simulink model "Correlation_Ex4"  (R2025a)
settings: Solver=VariableStepAuto  StartTime=0.0  StopTime=1024/100e6  RelTol=1e-3
undefined symbols (not defined in the file): Correlation_ValidMode, DUT, S, Valid, vsva2197, xcvc1902
libraries: visionstatistics x1, aieDSP x1, vmcUtilities x1
settings Model: Creator=sdegala  LastModifiedBy=robg
settings ModelReferenceCC: EnableRefExpFcnMdlSchedulingChecks=on
settings RTWCC: GPUComputeCapability=3.5

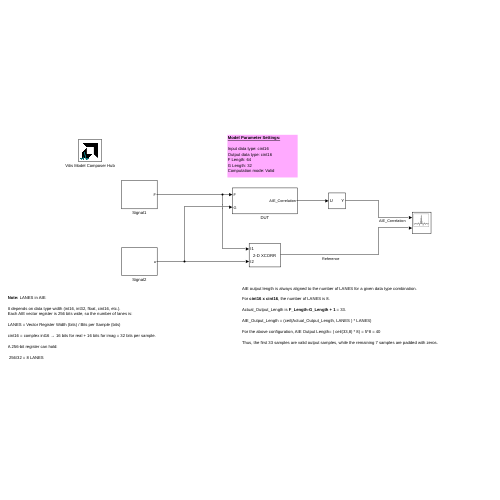
[thumbnail: Simulink's stored preview of the top-level diagram]
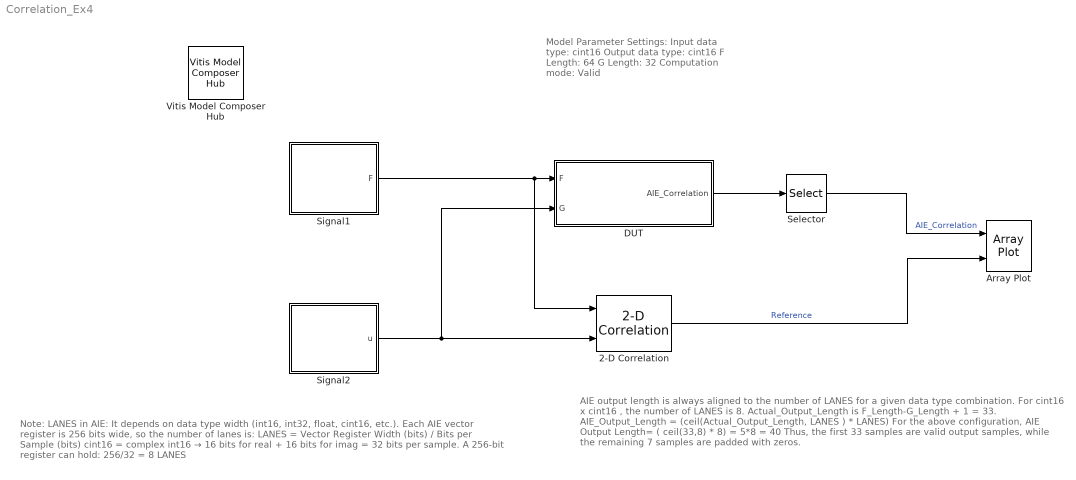
== system Correlation_Ex4 ==
  note: Note: LANES in AIE:
      |
      | It depends on data type width (int16, int32, float, cint16, etc.).
      | Each AIE vector register is 256 bits wide, so the number of lanes is:
      |
      | LANES = Vector Register Width (bits)​ / Bits per Sample (bits)
      |
      | cint16 = complex int16 → 16 bits for real + 16 bits for imag = 32 bits per sample.
      |
      | A 256-bit register can hold:
      |
      | 256/32 = 8 LANES
      |
      | ​
  note: AIE output length is always aligned to the number of LANES for a given data type combination.
      |
      | For cint16 x cint16 , the number of LANES is 8.
      |
      | Actual_Output_Length is F_Length-G_Length + 1 = 33.
      |
      | AIE_Output_Length = (ceil(Actual_Output_Length, LANES ) * LANES)
      |
      | For the above configuration, AIE Output Length= ( ceil(33,8) * 8) = 5*8 = 40
      |
      | Thus, the first 33 samples are valid output samples, while the remaining 7 samples are padded with zeros.
  note: Model Parameter Settings:
      |
      | Input data type: cint16
      | Output data type: cint16
      | F Length: 64
      | G Length: 32
      | Computation mode: Valid
  2-D Correlation : visionstatistics/2-D Correlation  outSize=Valid  normalize=off  roundingMode=Floor  overflowMode=off
  Array Plot : ArrayPlot  NumInputPorts=2  WindowPosition=[593.000000,365.000000,800.000000,500.000000,]  Visible=on  ScopeFrameLocation=window  YLimits=[-16.375 17.375]  ShowLegend=on
  DUT : Subsystem
  Selector : Selector  InputPortWidth=40  IndexOptions=Index vector (dialog)  Indices=1:1:64-(32-1)  OutputSizes=1
  Signal1 : Subsystem
  Signal2 : Subsystem
  Vitis Model Composer Hub : vmcUtilities/Vitis Model Composer Hub  Tag=genX  CodeGeneration=off  SubsystemName=DUT  BlockHierPath=Correlation_ValidMode/DUT  SubsystemType=AIENode  StartColumn=1  NumberOfColumns=1  TargetDirectory=./code  exportDesign=off  analyzeDesign=on  validateDesignOnHw=off  ExportType=AI Engines  IpVendor=xilinx.com  IpLibrary=hls  IpVersion=1.0  IpHWLanguage=Verilog  AieCompilerOptions={}  AieSimulatorOptions={}  CreateTestbench=on  TestbenchStackSize=10  RunRtlSim=off  RunCSim=off  RunAieSim=off  enableSimulationTimeout=on  enableGraphIterations=on  AieSimTimeout=50000  AieGraphIterations=-1  RunAieSimProfiling=off  LaunchVitisAnalyzer=off  PlotOutput=off  RunX86Sim=off  X86SimTimeout=10  GenHwImage=off  GenLibadfXo=off  GenHwValidationCode=off  PlatformType=Not Specified  HwSystemType=Baremetal  HwValidationTarget=hw  ProjDevice=xcvc1902-vsva2197-1LP-e-S  ProjDevicePart=xcvc1902-vsva2197-1LP-e-S  AIEType=AIE  SamplePeriod=-1  ClockFrequency=200  DataPathParallelism=1  xilinxfamily=versalaicore  part=xcvc1902  speed=-1LP-e-S  package=vsva2197  directory=./netlist  testbench=off  incr_netlist=off  synthesis_tool=Vivado  clock_wrapper=Clock Enables  dbl_ovrd=According to Block Masks  dcm_input_clock_period=10  sysclk_period=10  simulink_period=1  eval_field=0  IPInfoJsonString="{\"DUTSubsystemName\":\"DUT\",\"AIESubsystem\":{\"SubsystemName\":\"DUT\",\"TargetDirectory\":\"./code\",\"AIEArrayConfig\":\"Use entire AIE array\",\"StartColumn\":\"0\",\"NumberOfColumns\":\"1\"},\"SubsystemTag\":\"AIENode\"}"  LogFileName=/proj/xhdhdstaff5/sdegala/Head1/HEAD/2025_2_work/AIE_BLOCKS_2025_2/code/model_composer.log  NThreads=4  IPConfigFile=/tmp/vmctmp-11198269997411262707/Correlation_ValidMode_ipconfig.json
  wires:
  Signal2/1(u) -> 2-D Correlation/2, DUT/2(G)
  DUT/1(AIE_Correlation) -> Selector/1
  Signal1/1(F) -> DUT/1(F), 2-D Correlation/1
  2-D Correlation/1 -> Array Plot/2  "Reference"
  Selector/1 -> Array Plot/1  "AIE_Correlation"

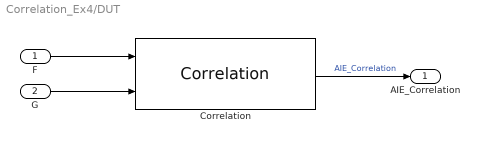
== system Correlation_Ex4/DUT ==
  F : Inport
  G : Inport  Port=2
  Correlation : aieDSP/Correlation  AIE_VARIANT=1  api=0  data_type_f=cint16  data_type_g=cint16  data_type_out=cint16  function_type=0  compute_mode=Valid (2)  f_sample_size=64  g_sample_size=32  USE_RTP_VECTOR_LENGTHS=off  num_frames=1  shift_output=0  rnd_mode=Floor  sat_mode=None  no_of_kernels=1  casc_length=1  blockJsonConstraints=[]  blockJsonConstraintsInternal=[]  spec=vmc_corr.json  SerializedMaskParamNames=[]  SerializedMaskParamValues=[]  SerializedMaskParamVisibilities=[]  block_type=Correlation  SerializedMaskParamDataypes=uint|uint|typename|typename|typename|uint|uint|uint|uint|uint|uint|uint|uint|uint|uint|uint  SerializedMaskParamEnumStrArr=0|0|0|0|0|0|Full (0),Same (1),Valid (2)|0|0|0|0|0|Floor,Ceiling,Round to positive infinity,Round to negative infinity,Round symmetrical to infinity,Round symmetrical to zero,Round convergent to even,Round convergent to odd|None,Saturate,Symmetric|0|0  SerializedMaskParamEnumValArr=0|0|0|0|0|0|0,1,2|0|0|0|0|0|0,1,2,3,4,5,6,7|0,1,3|0|0  SerializedMaskParamVectorArr=0|0|0|0|0|0|0|0|0|0|0|0|0|0|0|0  SerializedMaskParamKeys=AIE_VARIANT|TP_API|TT_DATA_F|TT_DATA_G|TT_DATA_OUT|TP_FUNCT_TYPE|TP_COMPUTE_MODE|TP_F_LEN|TP_G_LEN|TP_USE_RTP_VECTOR_LENGTHS|TP_NUM_FRAMES|TP_SHIFT|TP_RND|TP_SAT|TP_PHASES|TP_CASC_LEN
  AIE_Correlation : Outport
  wires:
  F/1 -> Correlation/1
  G/1 -> Correlation/2
  Correlation/1 -> AIE_Correlation/1  "AIE_Correlation"

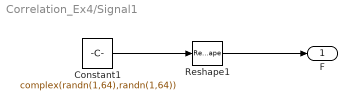
== system Correlation_Ex4/Signal1 ==
  Constant1 : Constant  Value=complex(randn(1,64),randn(1,64))  OutDataTypeStr=int16  SampleTime=1/100e6
  Reshape1 : Reshape
  F : Outport
  wires:
  Reshape1/1 -> F/1
  Constant1/1 -> Reshape1/1

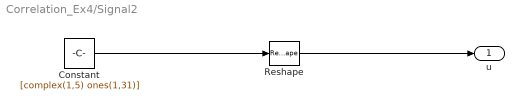
== system Correlation_Ex4/Signal2 ==
  Constant : Constant  Value=[complex(1,5) ones(1,31)]  OutDataTypeStr=int16  SampleTime=1/100e6
  Reshape : Reshape
  u : Outport
  wires:
  Reshape/1 -> u/1
  Constant/1 -> Reshape/1
